simulink model "diabetes_1step"  (R2022b)
settings: Solver=ode45  StartTime=0.0  StopTime=24  RelTol=1e-3  EnableMultiTasking=on
StopFcn:
  | step_results
libraries: simulink x2, realtime_pacer_lib x1
settings Model: Creator=tsladeche  LastModifiedBy=apple
settings SolverCC: AlgebraicLoopSolver=TrustRegion
settings DataIOCC: LimitDataPoints=on  SaveFormat=Array  SignalLoggingSaveFormat=ModelDataLogs  ReturnWorkspaceOutputs=off
settings OptimizationCC: ExpressionDepthLimit=2147483647  LifeSpan=inf
settings DebuggingCC: UnderspecifiedInitializationDetection=Classic  MergeDetectMultiDrivingBlocksExec=none  SolverPrmCheckMsg=warning  FcnCallInpInsideContextMsg=warning  UnconnectedInputMsg=warning  UnconnectedOutputMsg=warning  UnconnectedLineMsg=warning  StateNameClashWarn=warning  SFUnexpectedBacktrackingDiag=warning  SFNoUnconditionalDefaultTransitionDiag=warning  SFExecutionAtInitializationDiag=none  SFMachineParentedDataDiag=warning  ArithmeticOperatorsInVariantConditions=warning
settings HardwareCC: ProdBitPerPointer=32  ProdBitPerSizeT=32  ProdBitPerPtrDiffT=32  ProdLargestAtomicFloat=None  ProdIntDivRoundTo=Undefined  ProdEndianess=Unspecified  ProdWordSize=32  ProdHWDeviceType=32-bit Generic
settings ModelReferenceCC: PropagateSignalLabelsOutOfModel=off
settings SFSimCC: SimUseLocalCustomCode=off  CustomCodeUndefinedFunction=UseInterfaceOnly
settings RTWCC: RTWUseLocalCustomCode=off
settings CodeAppCC: StateflowObjectComments=on
settings GRTTargetCC: TargetLangStandard=C89/C90 (ANSI)  CombineOutputUpdateFcns=off  GRTInterface=on
settings ConfigComp: CovMetricSettings=dw  CovSaveCumulativeToWorkspaceVar=on  CovSaveSingleToWorkspaceVar=on  CovExternalEMLEnable=off

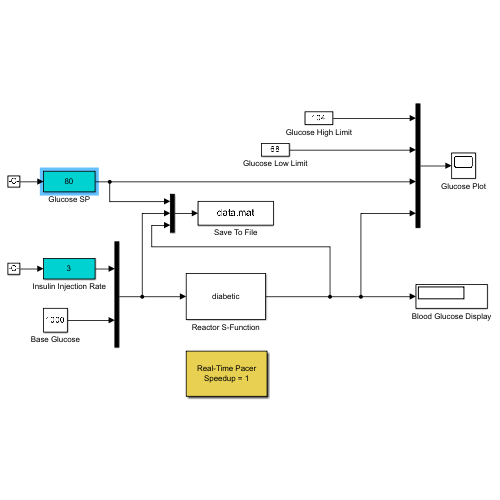
[thumbnail: Simulink's stored preview of the top-level diagram]
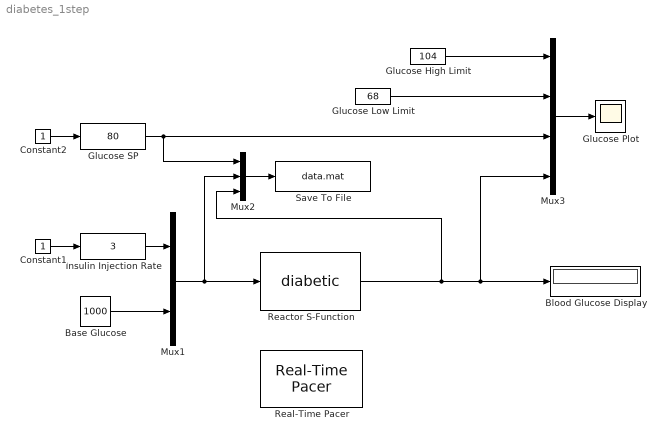
== system diabetes_1step ==
  Base Glucose : Constant  Value=1000
  Blood Glucose Display : Display
  Constant1 : Constant
  Constant2 : Constant
  Glucose High Limit : Constant  Value=104
  Glucose Low Limit : Constant  Value=68
  Glucose Plot : Scope
  Glucose SP : simulink/Math Operations/Slider Gain  gain=80  low=50  high=120
  Insulin Injection Rate : simulink/Math Operations/Slider Gain  gain=3  low=0  high=10
  Mux1 : Mux  Inputs=2
  Mux2 : Mux  Inputs=3
  Mux3 : Mux
  Reactor S-Function : S-Function  FunctionName=diabetic  SFunctionDeploymentMode=off  EnableBusSupport=off
  Real-Time Pacer : realtime_pacer_lib/Real-Time Pacer  simTimePerRealTime=1
  Save To File : ToFile  Filename=data.mat  MatrixName=diabetic  SampleTime=0.05
  wires:
  Mux2/1 -> Save To File/1
  Constant1/1 -> Insulin Injection Rate/1
  Mux1/1 -> Mux2/2, Reactor S-Function/1
  Constant2/1 -> Glucose SP/1
  Glucose SP/1 -> Mux3/3, Mux2/1
  Reactor S-Function/1 -> Mux3/4, Blood Glucose Display/1, Mux2/3
  Glucose High Limit/1 -> Mux3/1
  Glucose Low Limit/1 -> Mux3/2
  Mux3/1 -> Glucose Plot/1
  Insulin Injection Rate/1 -> Mux1/1
  Base Glucose/1 -> Mux1/2
